simulink model "ECUACION_DIFERENCIAL"  (R2024b)
settings: Solver=VariableStepAuto  StartTime=0.0  StopTime=10.0  RelTol=1e-3
settings Model: Creator=RREYM  LastModifiedBy=RREYM

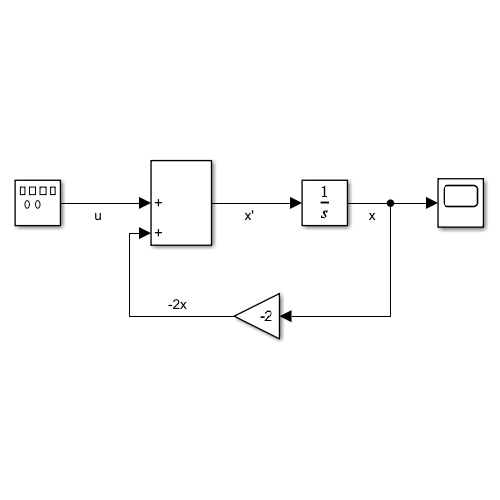
[thumbnail: Simulink's stored preview of the top-level diagram]
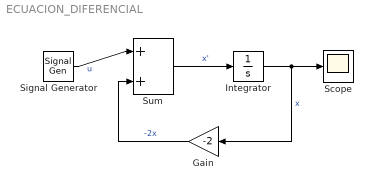
== system ECUACION_DIFERENCIAL ==
  Gain : Gain  Gain=-2
  Integrator : Integrator
  Scope : Scope
  Signal Generator : SignalGenerator  WaveForm=square  Units=rad/sec
  Sum : Sum  Inputs=|++
  wires:
  Signal Generator/1 -> Sum/1  "u"
  Sum/1 -> Integrator/1  "x'"
  Gain/1 -> Sum/2  "-2x"
  Integrator/1 -> Gain/1, Scope/1  "x"
